simulink model "week1_3"  (R2021a)
settings: Solver=VariableStepAuto  StartTime=0.0  StopTime=10.0  RelTol=1e-3
undefined symbols (not defined in the file): a0, a1, b1
settings Model: Creator=varunraj  LastModifiedBy=varunraj

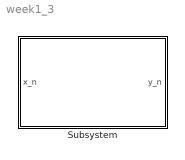
== system week1_3 ==
  Subsystem : Subsystem

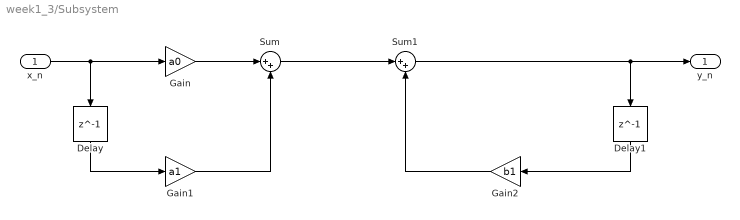
== system week1_3/Subsystem ==
  x_n : Inport
  Delay : Delay  DelayLength=1
  Delay1 : Delay  DelayLength=1
  Gain : Gain  Gain=a0
  Gain1 : Gain  Gain=a1
  Gain2 : Gain  Gain=b1
  Sum : Sum  Inputs=|++
  Sum1 : Sum  Inputs=|++
  y_n : Outport
  wires:
  x_n/1 -> Gain/1, Delay/1
  Delay/1 -> Gain1/1
  Gain/1 -> Sum/1
  Gain1/1 -> Sum/2
  Sum/1 -> Sum1/1
  Sum1/1 -> Delay1/1, y_n/1
  Delay1/1 -> Gain2/1
  Gain2/1 -> Sum1/2
